simulink model "Preprocesado"  (R2021b)
settings: Solver=VariableStepAuto  StartTime=0.0  StopTime=10.0  RelTol=1e-3
undefined symbols (not defined in the file): fdesignblkfcn, gcbh
libraries: dsparch4 x1
settings Model: Creator=alvaro  LastModifiedBy=alvaro

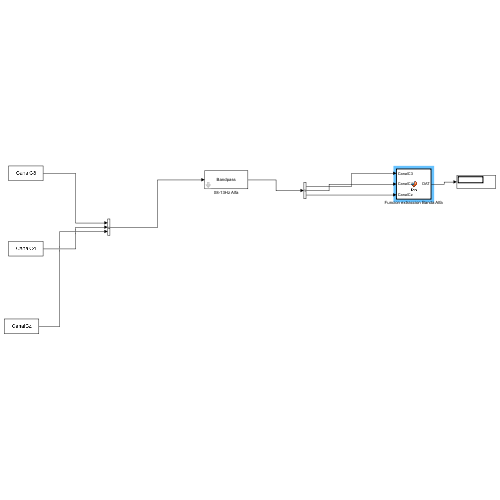
[thumbnail: Simulink's stored preview of the top-level diagram]
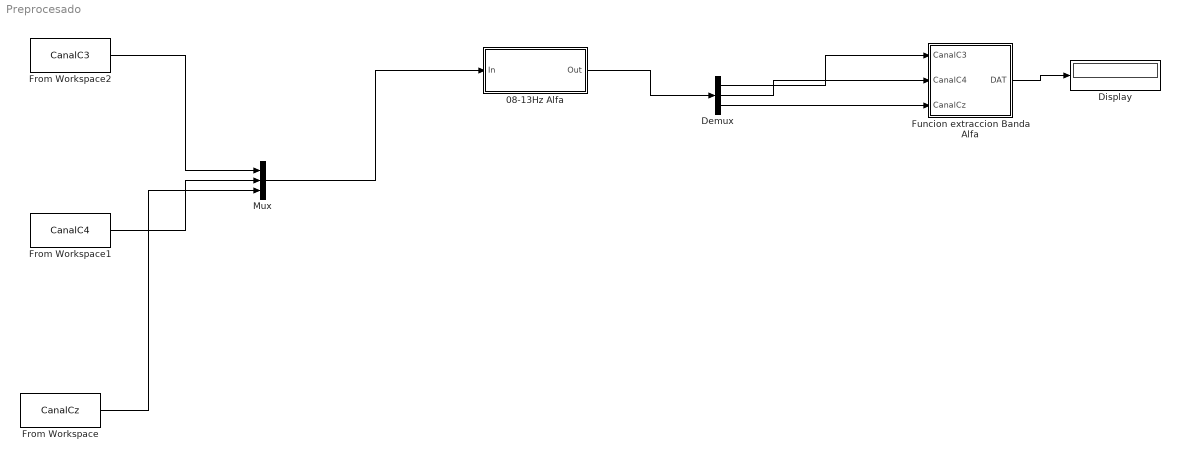
== system Preprocesado ==
  08-13Hz Alfa : Subsystem  DialogController=fdesignblkfcn  InitFcn=fdesignblkfcn(gcbh, {'InitFcn'});  mask(Bandpass Filter){}
      mask help: Design a bandpass filter
      settings: CopyFcn=fdesignblkfcn(gcbh, {'CopyFcn'});
      mask Help: helpview(mapfilelocation('dsp'), 'dspbandpassfilter');
      mask Display: disp('Bandpass');
  Demux : Demux  Outputs=3
      settings: DisplayOption=none
  Display : Display
  From Workspace : FromWorkspace  VariableName=CanalCz  SampleTime=160
  From Workspace1 : FromWorkspace  VariableName=CanalC4  SampleTime=160
  From Workspace2 : FromWorkspace  VariableName=CanalC3  SampleTime=160
  Funcion extraccion Banda Alfa : MATLAB Function  TreatAsAtomicUnit=on
  Mux : Mux  Inputs=3
  wires:
  Funcion extraccion Banda Alfa/1(DAT) -> Display/1
  From Workspace2/1 -> Mux/1
  From Workspace1/1 -> Mux/2
  From Workspace/1 -> Mux/3
  Mux/1 -> 08-13Hz Alfa/1(In)
  08-13Hz Alfa/1(Out) -> Demux/1
  Demux/1 -> Funcion extraccion Banda Alfa/1(CanalC3)
  Demux/3 -> Funcion extraccion Banda Alfa/3(CanalCz)
  Demux/2 -> Funcion extraccion Banda Alfa/2(CanalC4)

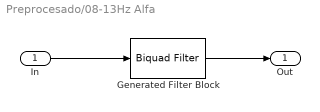
== system Preprocesado/08-13Hz Alfa ==
  In : Inport
  Generated Filter Block : dsparch4/Biquad Filter  Tag=BlockMethodSubSystem  FilterSource=Dialog parameters  CoeffSource=Specify via dialog  FilterObject=BQF  IIRFiltStruct=Direct form II  BiQuadCoeffs=[0.106193777977083598 0 -0.106193777977083598 1 -1.70817022912376837 0.836223107513699437;0.0287712784311114321 0 -0.0287712784311114321 1 -1.65259216844571899 0.816617541167721783;0.228933752509714789 0 -0.228933752509714789 1 -1.86379720464038678 0.961272776502518855;0.0557488790708176307 0 -0.0557488790708176307 1 -1.69650707415507318 0.940282353609846799;0.182028469565088447 0 -0.182028469565088447 1 -1.7845677565195861 0.890495241818041738;1.50270841788426179 0 -1.50270841788426179 1 -1.64361878317248067 0.850702967185112069]  ScaleValues=[0.0585193363851460036;1;1;1;1;1;1]  IC=0  ICnum=0  ICden=0  a0Flag=Warning  optimizeScaleValues=on  ScaleValueMode=Specify via input port (g)  roundingMode=Floor  overflowMode=off  scaleValueFracLength=14  denProdOutputFracLength=30  denAccumFracLength=30  secondMemoryFracLength=15
  Out : Outport
  wires:
  In/1 -> Generated Filter Block/1
  Generated Filter Block/1 -> Out/1

== matlab function Preprocesado/Funcion extraccion Banda Alfa ==
  settings: updateMethod=DISCRETE  sampleTime=160
  data: DAT output; CanalC3 input; CanalC4 input; CanalCz input
function DAT = fcn(CanalC3, CanalC4, CanalCz)
c3alfat=CanalC3;
czalfat=CanalCz;
c4alfat=CanalC4;
%Funcion Wavalet para descomponer la señas y tener reducir el nº de muestras
[cc3 ,lc3]= wavedec(c3alfat,2,'db2');
[ccz ,lcz]= wavedec(czalfat,2,'db2');
[cc4 ,lc4]= wavedec(c4alfat,2,'db2');
c3alfat = appcoef(cc3,lc3,'db2'); 
czalfat = appcoef(ccz,lcz,'db2'); 
c4alfat = appcoef(cc4,lc4,'db2'); 

%Calculamos la Densidad espectral de Potencia mediante el metodo Welch 
C3welchalfa = pwelch(c3alfat);
Czwelchalfa = pwelch(czalfat);
C4welchalfa= pwelch(c4alfat);

%Calculamos la FFT de la señal.
C3alfat = abs(fft(c3alfat)); 
Czalfat = abs(fft(czalfat));
C4alfat = abs(fft(c4alfat)); 

%%Extracion de Caracteristicas 
% Alfa 
C3VARa=var(C3alfat);
CzVARa=var(Czalfat);
C4VARa=var(C4alfat);
C3COVARa=cov(C3alfat);
CzCOVARa=cov(Czalfat);
C4COVARa=cov(C4alfat);
C3MEANa=cov(C3alfat);
CzMEANa=cov(Czalfat);
C4MEANa=cov(C4alfat);
C3STDa=std(C3alfat);
CzSTDa=std(Czalfat);
C4STDa=std(C4alfat);
C3MAXPSDa=max(C3welchalfa);
CzMAXPSDa=max(Czwelchalfa);
C4MAXPSDa=max(C4welchalfa);
c3VARa=var(c3alfat);
czVARa=var(czalfat);
c4VARa=var(c4alfat);
c3COVARa=cov(c3alfat);
czCOVARa=cov(czalfat);
c4COVARa=cov(c4alfat);
c3MEANa=cov(c3alfat);
czMEANa=cov(czalfat);
c4MEANa=cov(c4alfat);
c3STDa=std(c3alfat);
czSTDa=std(czalfat);
c4STDa=std(c4alfat);
c3MAXa=max(c3alfat);
czMAXa=max(czalfat);
c4MAXa=max(c4alfat);
c3MINa=min(c3alfat);
czMINa=min(czalfat);
c4MINa=min(c4alfat);

%Vector de caracteristicas 
DAT = [ C3VARa,C3COVARa,C3MEANa,C3STDa,C3MAXPSDa,c3VARa,c3COVARa,c3MEANa,c3STDa,c3MAXa,c3MINa,CzVARa,CzCOVARa,CzMEANa,CzMAXPSDa,CzSTDa,czVARa,czCOVARa,czMEANa,czSTDa,czMAXa,czMINa,C4VARa,C4COVARa,C4MEANa,C4MAXPSDa,C4STDa,c4VARa,c4COVARa,c4MEANa,c4STDa,c4MAXa,c4MINa];
